simulink model "pose_test_R2022b"  (R2022b)
settings: Solver=VariableStepAuto  StartTime=0.0  StopTime=1  RelTol=1e-3
libraries: robotgazebolib x3
settings Model: LastModifiedBy=22546723@sun.ac.za
settings OptimizationCC: ReuseModelBlockBuffer=on

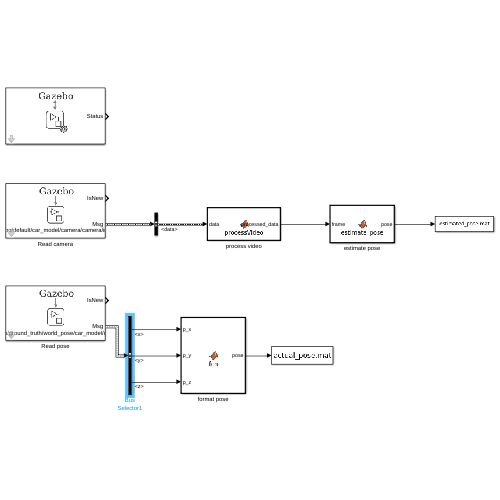
[thumbnail: Simulink's stored preview of the top-level diagram]
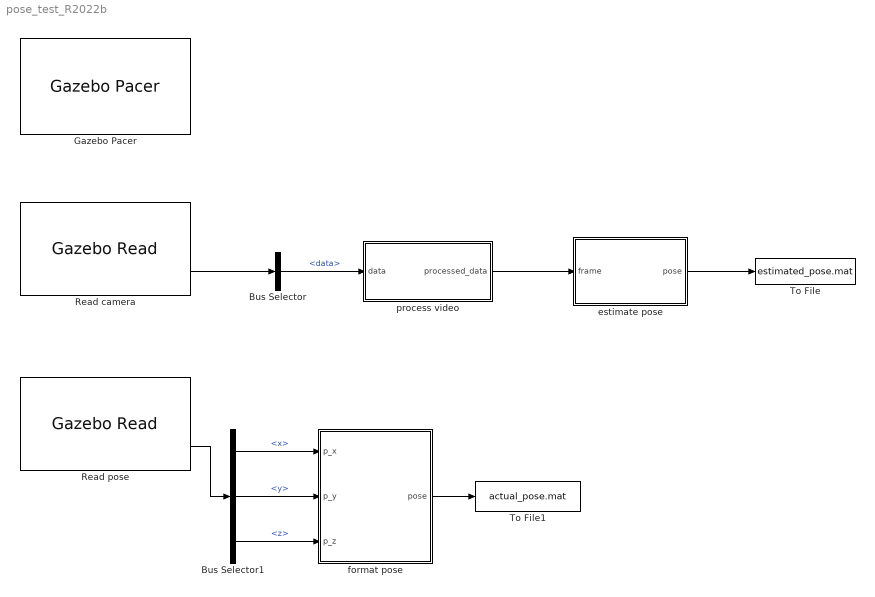
== system pose_test_R2022b ==
  Bus Selector : BusSelector  OutputSignals=data
  Bus Selector1 : BusSelector  OutputSignals=position.x,position.y,position.z
  Gazebo Pacer : robotgazebolib/Gazebo Pacer  ResetBehavior=Reset Gazebo simulation time  SampleTime=0.001
  Read camera : robotgazebolib/Gazebo Read  topicSource=From Gazebo  topic=/gazebo/default/car_model/camera/camera/image  messageType=gazebo_msgs/Image  sampleTime=0.001  fixedAxisBusStatus=off  jointAxisCount=2
  Read pose : robotgazebolib/Gazebo Read  topicSource=From Gazebo  topic=/gazebo/ground_truth/world_pose/car_model/camera  messageType=gazebo_msgs/Pose  sampleTime=0.001  fixedAxisBusStatus=off  jointAxisCount=2
  To File : ToFile  Filename=estimated_pose.mat  MatrixName=estimated_pose
  To File1 : ToFile  Filename=actual_pose.mat  MatrixName=actual_pose
  estimate pose : MATLAB Function  TreatAsAtomicUnit=on
  format pose : MATLAB Function  TreatAsAtomicUnit=on
  process video : MATLAB Function  TreatAsAtomicUnit=on
  wires:
  Read camera/2 -> Bus Selector/1
  Bus Selector/1 -> process video/1(data)  "<data>"
  Read pose/2 -> Bus Selector1/1
  process video/1(processed_data) -> estimate pose/1(frame)
  estimate pose/1(pose) -> To File/1
  format pose/1(pose) -> To File1/1
  Bus Selector1/1 -> format pose/1(p_x)  "<x>"
  Bus Selector1/2 -> format pose/2(p_y)  "<y>"
  Bus Selector1/3 -> format pose/3(p_z)  "<z>"

== matlab function pose_test_R2022b/estimate pose ==
  data: frame input; pose output
function pose = estimate_pose(frame)
coder.extrinsic('estimate');

poseEstimator = pose_estimator;
pose = zeros(4, 1, 1, 'double');
pose = estimate(poseEstimator, frame);

== matlab function pose_test_R2022b/process video ==
  data: data input; processed_data output
function processed_data=processVideo(data)
% the camera sends a 1200*600*3 data signal. Simulink receives it as a 1-D
% array

width = 1200;
height = 600;
z = 3;

processed_data = zeros(height, width, z, 'uint8');

if ~isempty(data) && ~isscalar(data)

    indexBase = (1:z:width*height*z)';
    index = zeros(numel(indexBase), z);

    for i=1:z
        index(:, i) = indexBase + i - 1;
    end

    temp = reshape(data(index), width, height, z);
    processed_data = permute(temp, [2 1 3]);

end

== matlab function pose_test_R2022b/format pose ==
  data: p_x input; pose output; p_y input; p_z input
function pose = fcn(p_x, p_y, p_z)
pose = [p_x p_y p_z];
